simulink model "blockScheme"  (R2022b)
settings: Solver=VariableStepAuto  StartTime=0.0  StopTime=30  RelTol=1e-3
libraries: slpidlib x1
settings Model: Creator=marak  LastModifiedBy=marak

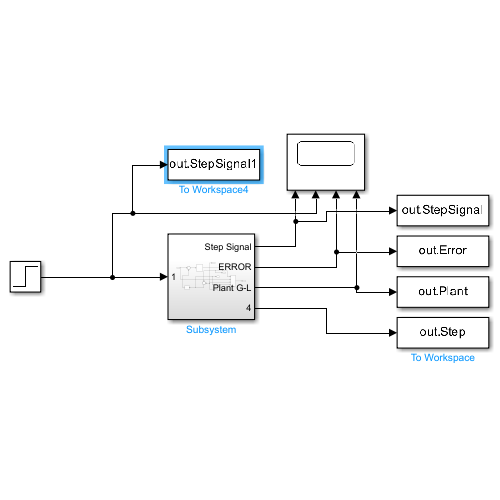
[thumbnail: Simulink's stored preview of the top-level diagram]
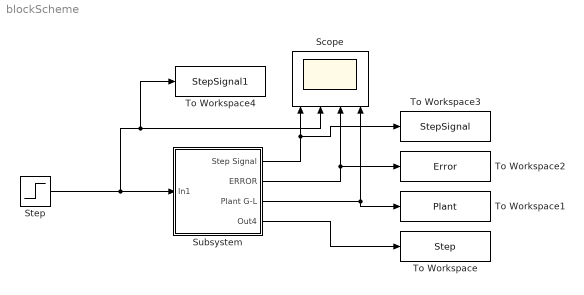
== system blockScheme ==
  Scope : Scope  NumInputPorts=4
  Step : Step  Time=14  After=0.3  SampleTime=0
  Subsystem : Subsystem
  To Workspace : ToWorkspace  VariableName=Step  SaveFormat=Timeseries  SampleTime=-1
  To Workspace1 : ToWorkspace  VariableName=Plant  SaveFormat=Timeseries  SampleTime=-1
  To Workspace2 : ToWorkspace  VariableName=Error  SaveFormat=Timeseries  SampleTime=-1
  To Workspace3 : ToWorkspace  VariableName=StepSignal  SaveFormat=Timeseries  SampleTime=-1
  To Workspace4 : ToWorkspace  VariableName=StepSignal1  SaveFormat=Timeseries  SampleTime=-1
  wires:
  Step/1 -> Subsystem/1(In1), To Workspace4/1, Scope/2
  Subsystem/1(Step Signal) -> Scope/1, To Workspace3/1
  Subsystem/2(ERROR) -> Scope/3, To Workspace2/1
  Subsystem/3(Plant G-L) -> Scope/4, To Workspace1/1
  Subsystem/4(Out4) -> To Workspace/1

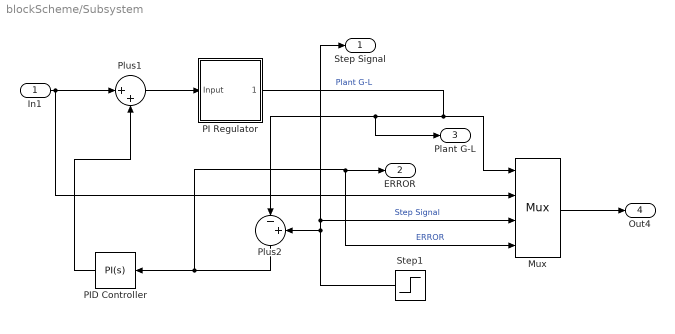
== system blockScheme/Subsystem ==
  In1 : Inport
  Mux : Mux
  PI Regulator : Subsystem  mask{m=1, k=1, b=2}
  PID Controller : slpidlib/PID Controller  Controller=PI  Form=Parallel  TimeDomain=Continuous-time  UseExternalTs=off  SampleTime=-1  IntegratorMethod=Forward Euler  FilterMethod=Forward Euler  ControllerParametersSource=internal  P=1.809  I=1.493  UseKiTs=off  D=0  N=100  UseFilter=on  TunerSelectOption=Transfer Function Based (PID Tuner App)  InitialConditionSource=internal  InitialConditionForIntegrator=0  InitialConditionForFilter=0  DifferentiatorICPrevScaledInput=0  ExternalReset=none  TrackingMode=off  Kt=1  LimitOutput=off  SatLimitsSource=internal  UpperSaturationLimit=inf  LowerSaturationLimit=-inf  LinearizeAsGain=on  AntiWindupMode=none  Kb=1  LimitIntegrator=off  UpperIntegratorSaturationLimit=inf  LowerIntegratorSaturationLimit=-inf  POutMin=[]  POutMax=[]  IOutMin=[]  IOutMax=[]  DOutMin=[]  DOutMax=[]  NOutMin=[]  NOutMax=[]  SumOutMin=[]  SumOutMax=[]  SaturationOutMin=[]  SaturationOutMax=[]  PParamMin=[]  PParamMax=[]  IParamMin=[]  IParamMax=[]  DParamMin=[]  DParamMax=[]  NParamMin=[]  NParamMax=[]  KbParamMin=[]  KbParamMax=[]  KtParamMin=[]  KtParamMax=[]  KbOutMin=[]  KbOutMax=[]  KtOutMin=[]  KtOutMax=[]  IntegratorOutMin=[]  IntegratorOutMax=[]  FilterOutMin=[]  FilterOutMax=[]  SumI1OutMin=[]  SumI1OutMax=[]  SumI2OutMin=[]  SumI2OutMax=[]  SumI3OutMin=[]  SumI3OutMax=[]  SumI4OutMin=[]  SumI4OutMax=[]  SumDOutMin=[]  SumDOutMax=[]  DifferentiatorOutMin=[]  DifferentiatorOutMax=[]  FilterDiffOutCoefMin=[]  FilterDiffOutCoefMax=[]  ReciprocalOutMin=[]  ReciprocalOutMax=[]  SumDenOutMin=[]  SumDenOutMax=[]  SumNumOutMin=[]  SumNumOutMax=[]  DivideOutMin=[]  DivideOutMax=[]  UdiffTsProdOutMin=[]  UdiffTsProdOutMax=[]  NTsProdOutMin=[]  NTsProdOutMax=[]  UintegralTsProdOutMin=[]  UintegralTsProdOutMax=[]  UngainTsProdOutMin=[]  UngainTsProdOutMax=[]  ClampingZeroOutDataTypeStr=Inherit: Inherit via back propagation  ClampingZeroOutMin=[]  ClampingZeroOutMax=[]  FilterDenConstantOutDataTypeStr=Inherit: Inherit via back propagation  FilterDenConstantOutMin=[]  FilterDenConstantOutMax=[]  PCopyOutDataTypeStr=Inherit: Inherit via back propagation  PCopyOutMin=[]  PCopyOutMax=[]  NCopyOutDataTypeStr=Inherit: Inherit via back propagation  NCopyOutMin=[]  NCopyOutMax=[]  IntegratorContinuousStateAttributes=''  IntegratorStateMustResolveToSignalObject=off  IntegratorRTWStateStorageClass=Auto  FilterContinuousStateAttributes=''  FilterStateMustResolveToSignalObject=off  FilterRTWStateStorageClass=Auto  ParallelPVariant=InternalParameters  IdealPVariant=Disabled  IVariant=InternalParameters  DVariant=Disabled  IntegratorVariant=Continuous  SatVariant=Disabled  AWVariant=Passthrough  PCopyVariant=Disabled  TRVariant=Disabled  FdbkBlocksVariant=Forward  IdealPFdbkVariant=Disabled  SatFdbkVariant=Disabled  DerivativeFilterVariant=Disabled  NVariant=Disabled  NCopyVariant=Disabled_SignalSpec  FilterICVariant=Disabled  IntegratorICVariant=InternalICs  ExternalResetVariant=Disabled  TRSumVariant=Passthrough  SumFdbkVariant=Disabled  SumVariant=Sum_PI  TsampFilterVariant=InternalTs  TsampNgainVariant=Passthrough  TsampIntegralVariant=Passthrough  ExternalSaturationOutDataTypeStr=Inherit: Same as second input
  Plus1 : Sum  Inputs=|++
  Plus2 : Sum  Inputs=|-+
  Step1 : Step  Time=10  Before=1  After=1.3  SampleTime=0
  Step Signal : Outport
  ERROR : Outport  Port=2
  Plant G-L : Outport  Port=3
  Out4 : Outport  Port=4
  wires:
  Step1/1 -> Mux/3, Step Signal/1, Plus2/2  "Step Signal"
  PID Controller/1 -> Plus1/2
  Plus2/1 -> ERROR/1, Mux/4, PID Controller/1  "ERROR"
  Plus1/1 -> PI Regulator/1(Input)
  Mux/1 -> Out4/1
  PI Regulator/1(Output) -> Plant G-L/1, Plus2/1, Mux/1  "Plant G-L"
  In1/1 -> Mux/2, Plus1/1

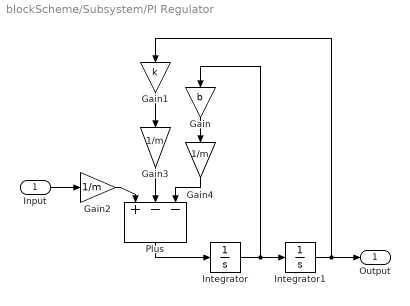
== system blockScheme/Subsystem/PI Regulator ==
  Input : Inport
  Gain : Gain  Gain=b
  Gain1 : Gain  Gain=k
  Gain2 : Gain  Gain=1/m
  Gain3 : Gain  Gain=1/m
  Gain4 : Gain  Gain=1/m
  Integrator : Integrator
  Integrator1 : Integrator
  Plus : Sum  Inputs=+--
  Output : Outport
  wires:
  Gain/1 -> Gain4/1
  Integrator1/1 -> Gain1/1, Output/1
  Integrator/1 -> Gain/1, Integrator1/1
  Gain1/1 -> Gain3/1
  Input/1 -> Gain2/1
  Plus/1 -> Integrator/1
  Gain3/1 -> Plus/2
  Gain2/1 -> Plus/1
  Gain4/1 -> Plus/3
